simulink model "LCK_0112"  (R2018b)
settings: Solver=FixedStepDiscrete  StartTime=0.0  StopTime=inf  FixedStep=0.01  RelTol=1e-3
PostLoadFcn:
  | if any(exist('dsrtsu_mdlpostloadfcn', 'file') ~= 0), dsrtsu_mdlpostloadfcn('Execute', bdroot); end
values from neighbouring files (symbols this model uses):
  C_DEG2RAD = 0.0175    [LCK_Macro.sldd]
  C_KPH2MPS = 0.2778    [LCK_Macro.sldd]
  C_NEARZERO = 0.0001    [LCK_Macro.sldd]
  C_ONE = 1.0    [LCK_Macro.sldd]
  C_RAD2DEG = 57.2958    [LCK_Macro.sldd]
  C_ZERO = 0.0    [LCK_Macro.sldd]
  k_accel_pedal_pos_per_speed_x : value not decoded    [LCK_LogicPara.sldd]
  k_accel_pedal_pos_per_speed_z : value not decoded    [LCK_LogicPara.sldd]
  k_brake_suprress_hold = 1000.0    [LCK_LogicPara.sldd]
  k_driver_appl_torque_filt = 50.0    [LCK_LogicPara.sldd]
  k_driver_suppression_hold_time = 3000.0    [LCK_LogicPara.sldd]
  k_hands_on_wheel_hold_msec = 500.0    [LCK_LogicPara.sldd]
  k_hands_on_wheel_torque_hi = 0.2    [LCK_LogicPara.sldd]
  k_hands_on_wheel_torque_lo = 0.15    [LCK_LogicPara.sldd]
  k_handsoff_delay_cycles = 50.0    [LCK_LogicPara.sldd]
  k_handsoff_torq_Lo_CR = 0.3    [LCK_LogicPara.sldd]
  k_handson_delay_cycles = 5.0    [LCK_LogicPara.sldd]
  k_HighAccel_suppress_hold = 3000.0    [LCK_LogicPara.sldd]
  k_HLR_suprress_hold = 3000.0    [LCK_LogicPara.sldd]
  k_hs_StrAng_CR_threshold_z : value not decoded    [LCK_LogicPara.sldd]
  k_LC_Exit_Switch = 0.0    [LCK_LogicPara.sldd]
  k_LCG_Configured = 1.0    [LCK_LogicPara.sldd]
  k_LCK_A0_Rdy2Act_UseConst = 0.0    [LCK_LogicPara.sldd]
  k_LCK_A0Fac_ActSta : value not decoded    [LCK_CtrlPara.sldd]
  k_LCK_A0Fac_DrvStm : value not decoded    [LCK_CtrlPara.sldd]
  k_LCK_A0Shift_LftCurv : value not decoded    [LCK_CtrlPara.sldd]
  k_LCK_A0Shift_RgtCurv : value not decoded    [LCK_CtrlPara.sldd]
  k_LCK_A0Shift_StraLan = 0.0    [LCK_CtrlPara.sldd]
  k_LCK_A0ShiftFac_Dy_LftCurv : value not decoded    [LCK_CtrlPara.sldd]
  k_LCK_A0ShiftFac_Dy_RgtCurv : value not decoded    [LCK_CtrlPara.sldd]
  k_LCK_A0ShiftFac_Vspd : value not decoded    [LCK_CtrlPara.sldd]
  k_LCK_accel_inhibit_thold = 35.0    [LCK_LogicPara.sldd]
  k_LCK_Active2Ready_Mask = 255.0    [LCK_LogicPara.sldd]
  k_LCK_CvatRateBks : value not decoded    [LCK_CtrlPara.sldd]
  k_LCK_CvatrBks : value not decoded    [LCK_CtrlPara.sldd]
  k_LCK_DFac_Dy : value not decoded    [LCK_CtrlPara.sldd]
  k_LCK_DFac_Dy_Curv : value not decoded    [LCK_CtrlPara.sldd]
  k_LCK_DFac_HaCurCen : value not decoded    [LCK_CtrlPara.sldd]
  k_LCK_DFac_HaCurSid : value not decoded    [LCK_CtrlPara.sldd]
  k_LCK_DFac_HadCurCen : value not decoded    [LCK_CtrlPara.sldd]
  k_LCK_DFac_HadCurSid : value not decoded    [LCK_CtrlPara.sldd]
  k_LCK_DFac_HadStrCen : value not decoded    [LCK_CtrlPara.sldd]
  k_LCK_DFac_HadStrSid : value not decoded    [LCK_CtrlPara.sldd]
  k_LCK_DFac_HaStrCen : value not decoded    [LCK_CtrlPara.sldd]
  k_LCK_DFac_HaStrSid : value not decoded    [LCK_CtrlPara.sldd]
  k_LCK_DFac_Rad : value not decoded    [LCK_CtrlPara.sldd]
  k_LCK_DFac_SA_CurCen : value not decoded    [LCK_CtrlPara.sldd]
  k_LCK_DFac_SA_CurSid : value not decoded    [LCK_CtrlPara.sldd]
  k_LCK_DFac_SA_StrCen : value not decoded    [LCK_CtrlPara.sldd]
  k_LCK_DFac_SA_StrSid : value not decoded    [LCK_CtrlPara.sldd]
  k_LCK_DFac_SS_CurCen : value not decoded    [LCK_CtrlPara.sldd]
  k_LCK_DFac_SS_CurSid : value not decoded    [LCK_CtrlPara.sldd]
  k_LCK_DFac_SS_StrCen : value not decoded    [LCK_CtrlPara.sldd]
  k_LCK_DFac_SS_StrSid : value not decoded    [LCK_CtrlPara.sldd]
  k_LCK_DFac_Vspd : value not decoded    [LCK_CtrlPara.sldd]
  k_LCK_DlyTm_DrvStim = 0.2    [LCK_CtrlPara.sldd]
  k_LCK_DTermMax = 2.0    [LCK_CtrlPara.sldd]
  k_LCK_DyBks_Curv : value not decoded    [LCK_CtrlPara.sldd]
  k_LCK_Enable_POOnly = 1.0    [LCK_LogicPara.sldd]
  k_LCK_Entry_DistBuffer = 0.1    [LCK_LogicPara.sldd]
  k_LCK_Fac_Vspd2RngThr_FalRec = 0.23    [LCK_CtrlPara.sldd]
  k_LCK_Ffw_CvatSwh = 0.0    [LCK_CtrlPara.sldd]
  k_LCK_Ffw_DyBks : value not decoded    [LCK_CtrlPara.sldd]
  k_LCK_Ffw_TimCon_CmdFlt = 0.0    [LCK_CtrlPara.sldd]
  k_LCK_FfwDeltaFac_Rad_Lft : value not decoded    [LCK_CtrlPara.sldd]
  k_LCK_FfwDeltaFac_Rad_Rgt : value not decoded    [LCK_CtrlPara.sldd]
  k_LCK_FfwDeltaFac_Vspd : value not decoded    [LCK_CtrlPara.sldd]
  k_LCK_FfwFac_CvatRate_Lft : value not decoded    [LCK_CtrlPara.sldd]
  k_LCK_FfwFac_CvatRate_Rgt : value not decoded    [LCK_CtrlPara.sldd]
  k_LCK_FfwFac_Dy : value not decoded    [LCK_CtrlPara.sldd]
  k_LCK_FfwFac_Rad_Lft : value not decoded    [LCK_CtrlPara.sldd]
  k_LCK_FfwFac_Rad_Rgt : value not decoded    [LCK_CtrlPara.sldd]
  k_LCK_FfwFac_Vspd : value not decoded    [LCK_CtrlPara.sldd]
  k_LCK_FfwTorq_Cvat : value not decoded    [LCK_CtrlPara.sldd]
  k_LCK_HAFac_ActSta : value not decoded    [LCK_CtrlPara.sldd]
  k_LCK_HAFac_DrvStm : value not decoded    [LCK_CtrlPara.sldd]
  k_LCK_HaloTime = 2000.0    [LCK_LogicPara.sldd]
  k_LCK_HaloTime_Switch = 0.0    [LCK_LogicPara.sldd]
  k_LCK_HARFac_ActSta : value not decoded    [LCK_CtrlPara.sldd]
  k_LCK_HARFac_DrvStm : value not decoded    [LCK_CtrlPara.sldd]
  k_LCK_Hed_DyBks : value not decoded    [LCK_CtrlPara.sldd]
  k_LCK_HedAngDiffX : value not decoded    [LCK_CtrlPara.sldd]
  k_LCK_HedAngRateDiffX : value not decoded    [LCK_CtrlPara.sldd]
  k_LCK_HndsOnWhel_DlyTm_Idl2Rdy = 0.0    [LCK_LogicPara.sldd]
  k_LCK_host_veh_width = 1.86    [LCK_LogicPara.sldd]
  k_LCK_Idle2Ready_Mask = 239.0    [LCK_LogicPara.sldd]
  k_LCK_Junc_SusTime = 1.0    [LCK_LogicPara.sldd]
  k_LCK_KpKdDecSlopeLmt = 10.0    [LCK_CtrlPara.sldd]
  k_LCK_KpKdIncSlopeLmt = 5.0    [LCK_CtrlPara.sldd]
  k_LCK_Lat_Ctrl_DFac_Lft = 1.0    [LCK_CtrlPara.sldd]
  k_LCK_Lat_Ctrl_DFac_Rgt = 1.05    [LCK_CtrlPara.sldd]
  k_LCK_Lat_Ctrl_Kd = 0.8    [LCK_CtrlPara.sldd]
  k_LCK_Lat_Ctrl_Ki = 0.5    [LCK_CtrlPara.sldd]
  k_LCK_Lat_Ctrl_Kp = 0.7    [LCK_CtrlPara.sldd]
  k_LCK_Lat_Ctrl_Kp_NearGain = 0.7    [LCK_CtrlPara.sldd]
  k_LCK_Lat_Ctrl_PFac_Lft = 1.0    [LCK_CtrlPara.sldd]
  k_LCK_Lat_Ctrl_PFac_Rgt = 1.05    [LCK_CtrlPara.sldd]
  k_LCK_Lat_Ctrl_TimCon_CmdFlt = 5.0    [LCK_CtrlPara.sldd]
  k_LCK_Lat_DFac_Rad : value not decoded    [LCK_CtrlPara.sldd]
  k_LCK_Lat_DFac_SS_Cur : value not decoded    [LCK_CtrlPara.sldd]
  k_LCK_Lat_DFac_SS_Str : value not decoded    [LCK_CtrlPara.sldd]
  k_LCK_Lat_DFac_Vspd : value not decoded    [LCK_CtrlPara.sldd]
  k_LCK_Lat_DyBks : value not decoded    [LCK_CtrlPara.sldd]
  k_LCK_Lat_IFac_Rad : value not decoded    [LCK_CtrlPara.sldd]
  k_LCK_Lat_IFac_Vspd : value not decoded    [LCK_CtrlPara.sldd]
  k_LCK_Lat_ILmtFac_Dy_CurvLan : value not decoded    [LCK_CtrlPara.sldd]
  k_LCK_Lat_ILmtFac_Dy_StraLan : value not decoded    [LCK_CtrlPara.sldd]
  k_LCK_Lat_ILmtFac_Rad : value not decoded    [LCK_CtrlPara.sldd]
  k_LCK_Lat_ILmtFac_Rad_NearGain = 1.0    [LCK_CtrlPara.sldd]
  k_LCK_Lat_ILmtFac_Vspd_CurvLan : value not decoded    [LCK_CtrlPara.sldd]
  k_LCK_Lat_ILmtFac_Vspd_StraLan : value not decoded    [LCK_CtrlPara.sldd]
  k_LCK_Lat_ITermLmt_Dy = 1.0    [LCK_CtrlPara.sldd]
  k_LCK_Lat_KpKdDecSlopeLmt = 10.0    [LCK_CtrlPara.sldd]
  k_LCK_Lat_KpKdIncSlopeLmt = 10.0    [LCK_CtrlPara.sldd]
  k_LCK_Lat_PFac_Dy_InnLftCur : value not decoded    [LCK_CtrlPara.sldd]
  k_LCK_Lat_PFac_Dy_InnRgtCur : value not decoded    [LCK_CtrlPara.sldd]
  k_LCK_Lat_PFac_Dy_OutLftCur : value not decoded    [LCK_CtrlPara.sldd]
  k_LCK_Lat_PFac_Dy_OutRgtCur : value not decoded    [LCK_CtrlPara.sldd]
  k_LCK_Lat_PFac_Dy_Str : value not decoded    [LCK_CtrlPara.sldd]
  k_LCK_Lat_PFac_Rad : value not decoded    [LCK_CtrlPara.sldd]
  ... (+153 more)
undefined symbols (not defined in the file or in its folder): k_LCK_CurvBks, K_LCK_SPA0A1A2_LMRngCmp_y
libraries: LateralControl_fcns_lib x58, simulink x24
(part 14 of 45)

== system LCK_0112/Lateral_Control_Module/Steer_Path_Process/Subsystem1 ==
  Lin01_ExistProb_Low : Inport
  Lin02_ExistProb_Low : Inport  Port=2
  LCK_Mode : Inport  Port=3
  Constant29 : Constant  Value=4
  Delay5 : Delay  DelayLength=1  InitialCondition=0
  Logical Operator27 : Logic  AllPortsSameDT=off  OutDataTypeStr=boolean
  Logical Operator28 : Logic  AllPortsSameDT=off  OutDataTypeStr=boolean
  Relational Operator20 : RelationalOperator  Operator===  OutDataTypeStr=boolean  RndMeth=Simplest
  Lin01_Invalid : Outport
  Lin02_Invalid : Outport  Port=2
  wires:
  Lin02_ExistProb_Low/1 -> Logical Operator28/2
  Relational Operator20/1 -> Logical Operator28/1, Logical Operator27/2
  Constant29/1 -> Relational Operator20/2
  Delay5/1 -> Relational Operator20/1
  Logical Operator27/1 -> Lin01_Invalid/1
  Lin01_ExistProb_Low/1 -> Logical Operator27/1
  LCK_Mode/1 -> Delay5/1
  Logical Operator28/1 -> Lin02_Invalid/1

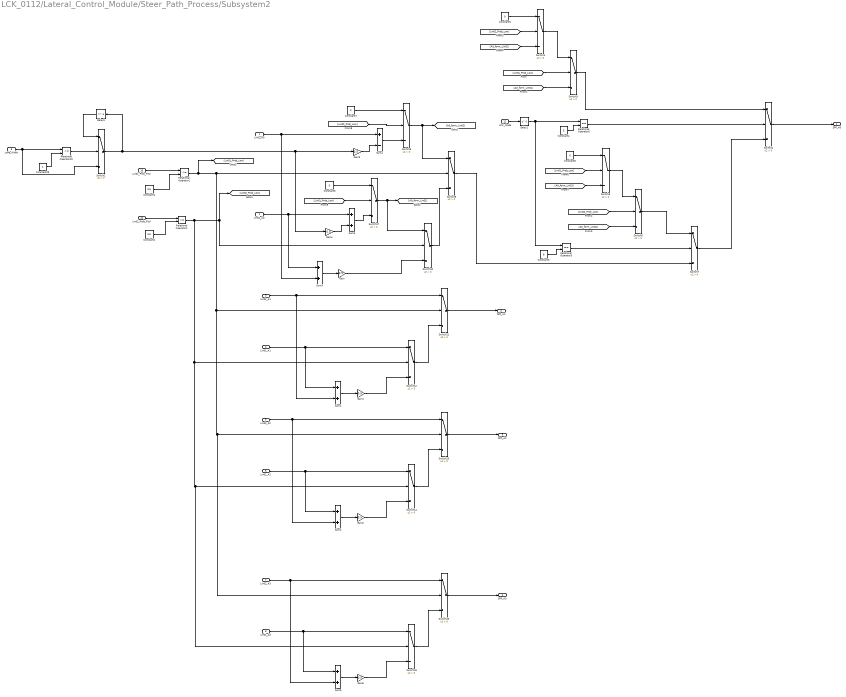
== system LCK_0112/Lateral_Control_Module/Steer_Path_Process/Subsystem2 ==
  Lin02_A0 : Inport
  Lin01_A0 : Inport  Port=2
  Lin02_A1 : Inport  Port=3
  Lin01_A1 : Inport  Port=4
  Lin02_A2 : Inport  Port=5
  Lin01_A2 : Inport  Port=6
  Lin02_A3 : Inport  Port=7
  Lin01_A3 : Inport  Port=8
  Lane_Width : Inport  Port=9
  Lin01_Prob_Fltd : Inport  Port=10
  Lin02_Prob_Fltd : Inport  Port=11
  LCK_Mode : Inport  Port=12
  Constant1 : Constant  Value=0.5
  Constant2 : Constant  Value=0.5
  Constant29 : Constant
  Constant3 : Constant  Value=6
  Constant4 : Constant  Value=5
  Constant{5..8} (4 alike) : Constant  Value=0
  Delay1 : Delay  DelayLength=1  InitialCondition=0
  Delay5 : Delay  DelayLength=1  InitialCondition=0
  Gain{,1..5} (6 alike) : Gain  Gain=0.5
  Relational Operator1 : RelationalOperator  Operator=<=  OutDataTypeStr=boolean  RndMeth=Simplest
  Relational Operator2 : RelationalOperator  Operator=<=  OutDataTypeStr=boolean  RndMeth=Simplest
  Relational Operator20 : RelationalOperator  Operator=<=  OutDataTypeStr=boolean  RndMeth=Simplest
  Relational Operator3 : RelationalOperator  Operator===  OutDataTypeStr=boolean  RndMeth=Simplest
  Relational Operator5 : RelationalOperator  Operator===  OutDataTypeStr=boolean  RndMeth=Simplest
  Sum{1..3,5..6} (5 alike) : Sum  Description=_GWMAB30P2.LCK.000_1362_  LockScale=on
  Sum4 : Sum  Description=_GWMAB30P2.LCK.000_1362_  Inputs=+-  LockScale=on
  Switch{1..17} (17 alike) : Switch  Criteria=u2 > Threshold
  SPP_A0 : Outport
  SPP_A1 : Outport  Port=2
  SPP_A2 : Outport  Port=3
  SPP_A3 : Outport  Port=4
  wires:
  Gain/1 -> Switch10/3
  Lin01_A1/1 -> Sum1/1, Switch12/1
  Lin02_A0/1 -> Sum3/2, Sum4/1
  Lin02_A1/1 -> Switch11/1, Sum1/2
  Gain4/1 -> Sum5/2
  Sum3/1 -> Gain/1
  Switch12/1 -> Switch11/3
  Gain3/1 -> Sum4/2
  Sum1/1 -> Gain1/1
  Gain1/1 -> Switch12/3
  Sum2/1 -> Gain2/1
  Switch14/1 -> Switch13/3
  Switch10/1 -> Switch9/3
  Switch16/1 -> Switch15/3
  Sum6/1 -> Gain5/1
  Gain2/1 -> Switch14/3
  Switch15/1 -> SPP_A3/1
  Gain5/1 -> Switch16/3
  Lin02_A3/1 -> Sum6/2, Switch15/1
  Lin01_A0/1 -> Sum3/1, Sum5/1
  Lin01_A2/1 -> Sum2/1, Switch14/1
  Lin02_A2/1 -> Sum2/2, Switch13/1
  Lin01_A3/1 -> Sum6/1, Switch16/1
  Switch11/1 -> SPP_A1/1
  Switch13/1 -> SPP_A2/1
  Constant29/1 -> Relational Operator20/2
  Lane_Width/1 -> Relational Operator20/1, Switch1/3
  Relational Operator20/1 -> Switch1/2
  Switch1/1 -> Gain3/1, Gain4/1, Delay5/1
  Delay5/1 -> Switch1/1
  Lin01_Prob_Fltd/1 -> Relational Operator1/1
  Constant1/1 -> Relational Operator1/2
  Relational Operator1/1 -> [Lin01_Prob_Low], Switch9/2, Switch15/2, Switch13/2, Switch11/2
  Lin02_Prob_Fltd/1 -> Relational Operator2/1
  Constant2/1 -> Relational Operator2/2
  Relational Operator2/1 -> Switch10/2, [Lin02_Prob_Low], Switch12/2, Switch16/2, Switch14/2
  Constant3/1 -> Relational Operator3/2
  Constant4/1 -> Relational Operator5/2
  LCK_Mode/1 -> Delay1/1
  Delay1/1 -> Relational Operator3/1, Relational Operator5/1
  Relational Operator5/1 -> Switch2/2
  [Lin01_Prob_Low] -> Switch3/2
  [A0_form_Lin01] -> Switch3/3
  [Lin02_Prob_Low] -> Switch4/2
  Constant5/1 -> Switch4/1
  [A0_form_Lin02] -> Switch4/3
  Switch4/1 -> Switch3/1
  Switch3/1 -> Switch2/1
  Switch6/1 -> Switch5/1
  [A0_form_Lin01] -> Switch6/3
  Constant6/1 -> Switch6/1
  [Lin01_Prob_Low] -> Switch6/2
  [A0_form_Lin02] -> Switch5/3
  [Lin02_Prob_Low] -> Switch5/2
  Switch5/1 -> Switch7/1
  Relational Operator3/1 -> Switch7/2
  Switch7/1 -> Switch2/3
  Switch2/1 -> SPP_A0/1
  Switch9/1 -> Switch7/3
  Sum4/1 -> Switch8/3
  [Lin02_Prob_Low] -> Switch8/2
  Constant7/1 -> Switch8/1
  Switch8/1 -> Switch9/1, [A0_form_Lin02]
  [Lin01_Prob_Low] -> Switch17/2
  Constant8/1 -> Switch17/1
  Sum5/1 -> Switch17/3
  Switch17/1 -> Switch10/1, [A0_form_Lin01]

== system LCK_0112/RTI Data/RTI Data Store/RTI Data Store ==
  RTI Data Store : Subsystem  mask(RTI_DATA_STORE){}
      mask help:
      | RTI Data Store Block. This block is used by RTI to store internal model dependent data. Deleting this block will result in data loss.
      |
      | NEVER DELETE, COPY, OR MODIFY THIS BLOCK!
      mask Help:
      | RTI Data Store Block. This block is used by RTI to store internal model dependent data. Deleting this block will result in data loss.
      | 
      | NEVER DELETE, COPY, OR MODIFY THIS BLOCK!
      mask Display: text(0.5, 0.5, ' ', 'HorizontalAlignment', 'center');
